simulink model "sgMdl_IO908_SharedMemoryLoopback"  (R2024b)
settings: Solver=FixedStepAuto  StartTime=0.0  StopTime=inf  RelTol=1e-3
undefined symbols (not defined in the file): Partitions
libraries: speedgoatlib_sharedmemory x7, slrealtimesharedmemorylib x4, simulink x1, speedgoatlib_interrupt x1
Description:
  | IO908 - Shared Memory Loopback
settings Model: ModifiedByFormat=Speedgoat  SimulationMode=external  ExtModeTrigDuration=100000  Creator=Speedgoat  LastModifiedBy=Speedgoat
settings SolverCC: ConcurrentTasks=on  PositivePriorityOrder=on
settings OptimizationCC: BlockReduction=off  OptimizeBlockIOStorage=off  ReuseModelBlockBuffer=off
settings DebuggingCC: TasksWithSamePriorityMsg=none
settings HardwareCC: ProdBitPerLong=64  ProdLongLongMode=on  ProdHWDeviceType=Intel->x86-64 (Linux 64)
settings RTWCC: Description=Speedgoat Real-Time Target Machine  SystemTargetFile=speedgoat.tlc  TemplateMakefile=slrealtime_default_tmf  Toolchain=Simulink Real-Time Toolchain  BuildConfiguration=Faster Runs  TargetLang=C++  GPUComputeCapability=3.5
settings SimulinkRealTimeTargetCC: SubcomponentCodeInterfacePackaging=Reusable function  InstructionSetFMA=off  LogToMDFFile=off  SLRTFileLogMaxRuns=10
settings ConfigComp: CovBoundaryAbsTol=1.0e-5

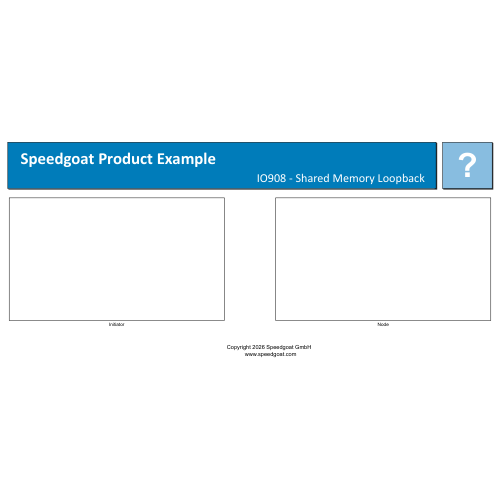
[thumbnail: Simulink's stored preview of the top-level diagram]
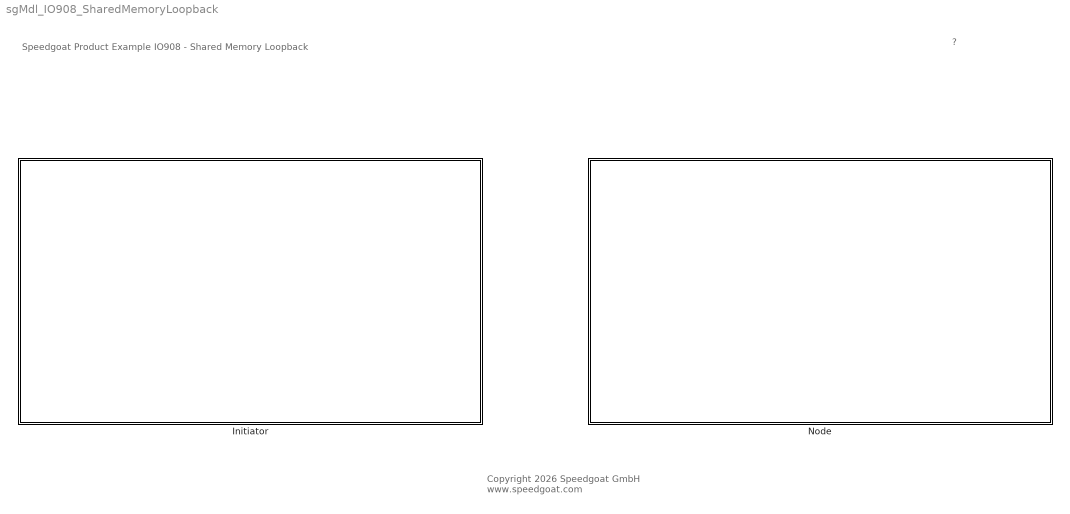
== system sgMdl_IO908_SharedMemoryLoopback ==
  note: Speedgoat Product Example
      | IO908 - Shared Memory Loopback
  note: ?
  note: Copyright 2026 Speedgoat GmbH
      |  www.speedgoat.com
  Initiator : Subsystem
  Node : Subsystem

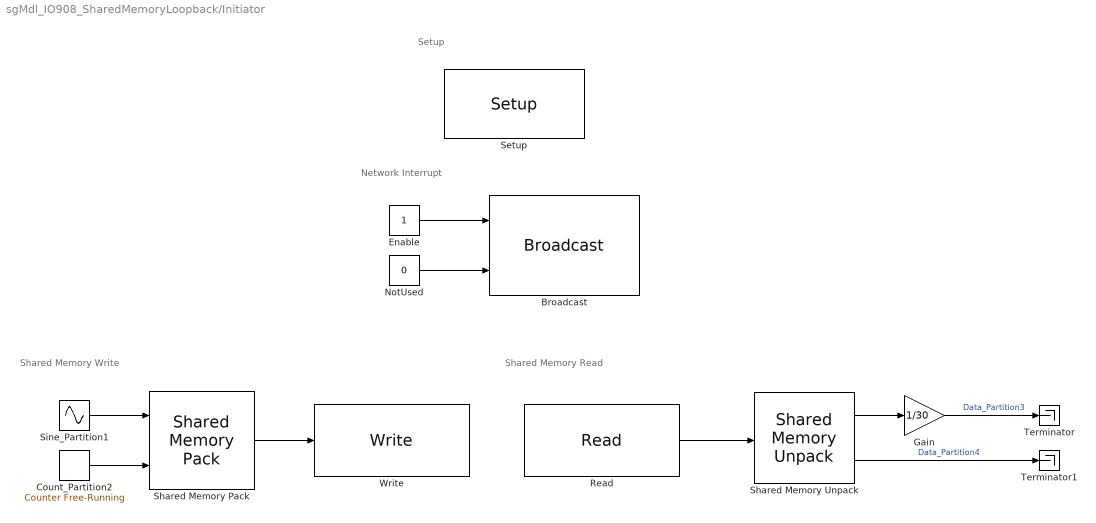
== system sgMdl_IO908_SharedMemoryLoopback/Initiator ==
  note: Network Interrupt
  note: Shared Memory Read
  note: Shared Memory Write
  note: Setup
  Broadcast : speedgoatlib_sharedmemory/Broadcast  moduleType=IO908  id=1  ninterrupt=1  target=-1  ts=-1  pci=-1
      settings: SourceProductName=Simulink Real-Time: Speedgoat I/O Blockset
      settings: AttributesFormatString=|
      | IRQ number = %<ninterrupt>
      | Target Node = %<target>
  Count_Partition2 : simulink/Sources/Counter Free-Running  NumBits=32  tsamp=0.001
  Enable : Constant  OutDataTypeStr=Inherit: Inherit via back propagation  SampleTime=0.001
  Gain : Gain  Gain=1/30
  NotUsed : Constant  Value=0  OutDataTypeStr=Inherit: Inherit via back propagation  SampleTime=0.001
  Read : speedgoatlib_sharedmemory/Read  moduleType=IO908  id=1  mode=Initiator  partition=[Partitions(3:4)]  ts=0.001  pci=-1  errport=off
      settings: SourceProductName=Simulink Real-Time: Speedgoat I/O Blockset
  Setup : speedgoatlib_sharedmemory/Setup  moduleType=IO908  id=1  node=node1  pci=-1
      settings: SourceProductName=Simulink Real-Time: Speedgoat I/O Blockset
  Shared Memory Pack : slrealtimesharedmemorylib/Shared Memory Pack  partition=[Partitions(1:2)]
      settings: AttributesFormatString=Partitions = %<partition>
  Shared Memory Unpack : slrealtimesharedmemorylib/Shared Memory Unpack  partition=[Partitions(3:4)]
      settings: AttributesFormatString=Partitions = %<partition>
  Sine_Partition1 : Sin  Amplitude=10  Frequency=2*pi  SampleTime=0.001
  Terminator : Terminator
  Terminator1 : Terminator
  "Write " : speedgoatlib_sharedmemory/Write   moduleType=IO908  id=1  partition=[Partitions(1:2)]  ts=-1  pci=-1  errport=off  enDMA=off
      settings: SourceProductName=Simulink Real-Time: Speedgoat I/O Blockset
  wires:
  Enable/1 -> Broadcast/1
  Shared Memory Pack/1 -> "Write "/1
  Read/1 -> Shared Memory Unpack/1
  NotUsed/1 -> Broadcast/2
  Count_Partition2/1 -> Shared Memory Pack/2
  Gain/1 -> Terminator/1  "Data_Partition3"
  Shared Memory Unpack/2 -> Terminator1/1  "Data_Partition4"
  Sine_Partition1/1 -> Shared Memory Pack/1
  Shared Memory Unpack/1 -> Gain/1

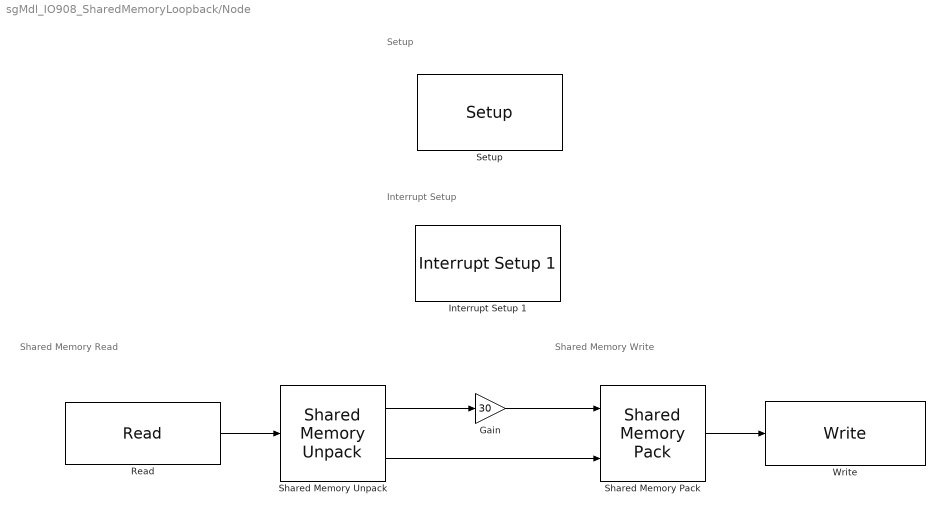
== system sgMdl_IO908_SharedMemoryLoopback/Node ==
  note: Setup
  note: Shared Memory Read
  note: Interrupt Setup
  note: Shared Memory Write
  Gain : Gain  Gain=30
  Interrupt Setup 1 : speedgoatlib_interrupt/Interrupt Setup 1  parModuleTrigger=on  parPollingMode=off  parPriorityConf=High  parPriority=241  confStartFcn=IO907_start_public  confStopFcn=IO907_stop_public  confIsrFcn=IO907_isr_public  confMapFcn=IO907_map_public  confHookFile=io907_int_hooks.c  confIrqNr=-1  confIsPolling=off  confModID=16776961  confSelectedInt=Speedgoat IO908 interrupt  confSelectedId=1  confSelectedChannel=[]  confData=[]  confForcePollingMode=off
  Read : speedgoatlib_sharedmemory/Read  moduleType=IO908  id=1  mode=Initiator  partition=[Partitions(1:2)]  ts=-1  pci=-1  errport=off
      settings: SourceProductName=Simulink Real-Time: Speedgoat I/O Blockset
  Setup : speedgoatlib_sharedmemory/Setup  moduleType=IO908  id=1  node=node2  pci=-1
      settings: SourceProductName=Simulink Real-Time: Speedgoat I/O Blockset
  Shared Memory Pack : slrealtimesharedmemorylib/Shared Memory Pack  partition=[Partitions(3:4)]
      settings: AttributesFormatString=Partitions = %<partition>
  Shared Memory Unpack : slrealtimesharedmemorylib/Shared Memory Unpack  partition=[Partitions(1:2)]
      settings: AttributesFormatString=Partitions = %<partition>
  "Write " : speedgoatlib_sharedmemory/Write   moduleType=IO908  id=1  partition=[Partitions(3:4)]  ts=-1  pci=-1  errport=off  enDMA=off
      settings: SourceProductName=Simulink Real-Time: Speedgoat I/O Blockset
  wires:
  Gain/1 -> Shared Memory Pack/1
  Shared Memory Pack/1 -> "Write "/1
  Shared Memory Unpack/2 -> Shared Memory Pack/2
  Read/1 -> Shared Memory Unpack/1
  Shared Memory Unpack/1 -> Gain/1
